simulink model "drone"  (R2019b)
settings: Solver=FixedStepAuto  StartTime=0.0  StopTime=10.0  FixedStep=0.5  RelTol=1e-3
model workspace (MAT data in the model file):
  UAVid = 0
undefined symbols (not defined in the file or in its folder): m, n
libraries: aerolibactuator x3
settings Model: ParameterArgumentNames=UAVid  OrderedModelArguments=off  Creator=Rafael.Casado  LastModifiedBy=paloma

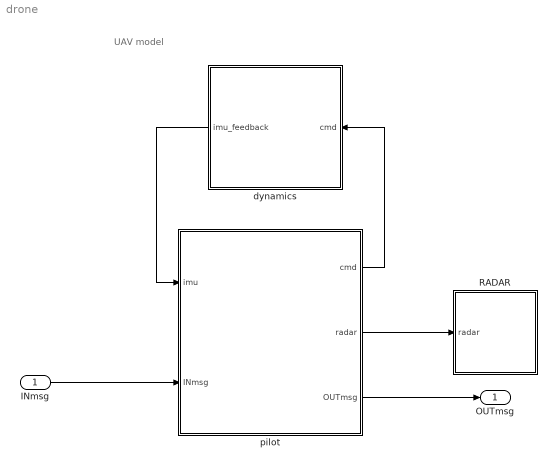
== system drone ==
  note: UAV model
  INmsg : Inport  OutputPortMessageModes=m  OutDataTypeStr=Bus: bus_msg  BusOutputAsStruct=on
  RADAR : Subsystem
      mask Display:
      | plot([00 10], [05 05])
      | plot([05 05], [00 10])
      | 
      | plot([01 09 09 01 01], [01 01 09 09 01])
      | plot([03 07 07 03 03], [03 03 07 07 03])
  dynamics : Subsystem
  pilot : Stateflow chart  TreatAsAtomicUnit=on
  OUTmsg : Outport  OutDataTypeStr=Bus: bus_msg  BusOutputAsStruct=on
  wires:
  pilot/2(radar) -> RADAR/1(radar)
  INmsg/1 -> pilot/2(INmsg)
  pilot/1(cmd) -> dynamics/1(cmd)
  pilot/3(OUTmsg) -> OUTmsg/1
  dynamics/1(imu_feedback) -> pilot/1(imu)

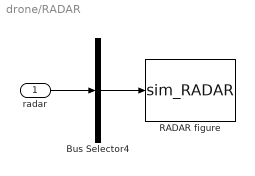
== system drone/RADAR ==
  radar : Inport
  Bus Selector4 : BusSelector  OutputSignals=id,x,y,z  OutputAsBus=on
  RADAR figure : MATLABFcn  StartFcn=|  MATLABFcn=sim_RADAR  OutputDimensions=0  Output1D=off
      | clear functions;
      | clc;
      mask Display: patch([50 -50 -50 50], [40 40 -60 -60], [1 1 1])
  wires:
  radar/1 -> Bus Selector4/1
  Bus Selector4/1 -> RADAR figure/1

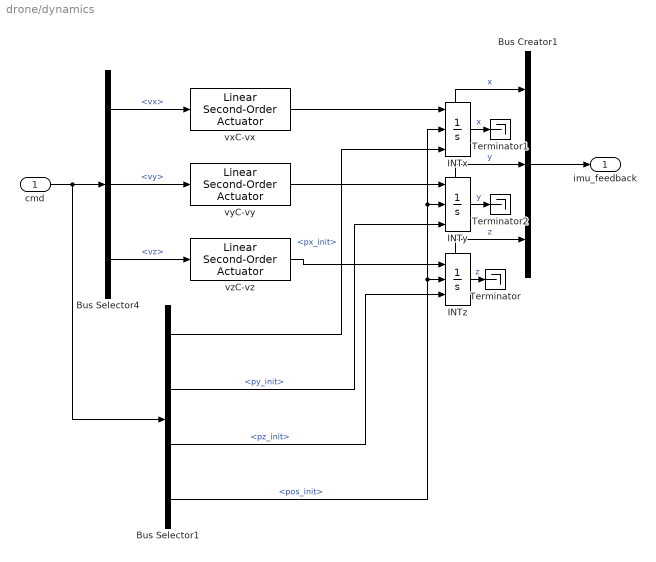
== system drone/dynamics ==
  cmd : Inport
  Bus Creator1 : BusCreator  Inputs=3  OutDataTypeStr=Bus: bus_IMU
      settings: InheritFromInputs=off
  Bus Selector1 : BusSelector  OutputSignals=px_init,py_init,pz_init,pos_init
  Bus Selector4 : BusSelector  OutputSignals=vx,vy,vz
  INTx : Integrator  ExternalReset=rising  InitialConditionSource=external  ShowStatePort=on
  INTy : Integrator  ExternalReset=rising  InitialConditionSource=external  ShowStatePort=on
  INTz : Integrator  ExternalReset=rising  InitialConditionSource=external  ShowStatePort=on
  Terminator : Terminator
  Terminator1 : Terminator
  Terminator2 : Terminator
  vxC-vx : aerolibactuator/Linear Second-Order Actuator  wn_fin=1  z_fin=0.3  fin_act_0=0  fin_act_vel=0
      settings: SourceProductName=Aerospace Blockset  SourceProductBaseCode=AE
  vyC-vy : aerolibactuator/Linear Second-Order Actuator  wn_fin=1  z_fin=0.3  fin_act_0=0  fin_act_vel=0
      settings: SourceProductName=Aerospace Blockset  SourceProductBaseCode=AE
  vzC-vz : aerolibactuator/Linear Second-Order Actuator  wn_fin=1  z_fin=0.3  fin_act_0=0  fin_act_vel=0
      settings: SourceProductName=Aerospace Blockset  SourceProductBaseCode=AE
  imu_feedback : Outport  SourceOfInitialOutputValue=Input signal  OutputWhenDisabled=reset  VectorParamsAs1DForOutWhenUnconnected=off
  wires:
  Bus Creator1/1 -> imu_feedback/1
  INTy/State -> Bus Creator1/2  "y"
  INTx/State -> Bus Creator1/1  "x"
  INTz/State -> Bus Creator1/3  "z"
  Bus Selector4/3 -> vzC-vz/1  "<vz>"
  Bus Selector4/1 -> vxC-vx/1  "<vx>"
  Bus Selector4/2 -> vyC-vy/1  "<vy>"
  vxC-vx/1 -> INTx/1
  vyC-vy/1 -> INTy/1
  vzC-vz/1 -> INTz/1
  Bus Selector1/1 -> INTx/3  "<px_init>"
  Bus Selector1/4 -> INTz/2, INTy/2, INTx/2  "<pos_init>"
  Bus Selector1/2 -> INTy/3  "<py_init>"
  cmd/1 -> Bus Selector1/1, Bus Selector4/1
  Bus Selector1/3 -> INTz/3  "<pz_init>"
  INTz/1 -> Terminator/1  "z"
  INTy/1 -> Terminator2/1  "y"
  INTx/1 -> Terminator1/1  "x"

== stateflow chart drone/pilot ==
  state NAVIGATOR [parallel]
    settings: executionOrder=1
    state INIT
      entry:
      initF
    state IDLE
      entry:
      idleF
    state TAKINGOFF
      entry:
      takingoffF
    state LANDING
      entry,during:
      landingF
    state FLYING
      entry, during:
      d = flyingF;
    (default) -> INIT
    INIT -> IDLE : [active]
    IDLE -> TAKINGOFF : [delivering]
    LANDING -> IDLE : [imu.z < 1]
    TAKINGOFF -> FLYING : [imu.z > 20]
    FLYING -> LANDING : [d<10]
  state COMUNICATIONS [parallel]
    updateRadar
    msgsProcess
    settings: executionOrder=2
    state msgsProcess [function]
      (default) -> (junction 143)
      (junction 143) -> (junction 138) [order 1] : INmsg
      (junction 145) -> (junction 143)
      (junction 143) -> (junction 139) [order 2]
      (junction 138) -> (junction 145) : {UAVmsgProcess}
  data: dis function_output; imu input Bus: bus_IMU; cmd output Bus: bus_command; INmsg input Bus: bus_msg; radar output Bus: bus_radar; OUTmsg output Bus: bus_msg; UAVid parameter double; delivering local boolean =false; deliverPos local; curTime local; d local; vto local =1; active local boolean =false
  function initF:
    | function initF
    | 
    | % Leo matriz de posiciones inicio UAVs (*AppDesign)
    | coder.extrinsic('evalin')
    | beginning = evalin('base','R2');
    | len = double(0);
    | len = length(beginning);
    | 
    | %Asigno posiciones de inicio 
    | if UAVid<=len
    |     active = true;
    |     cmd.pos_init = true;
    |     cmd.px_init  = beginning(UAVid,1);
    |     cmd.py_init  = beginning(UAVid,2);
    |     cmd.pz_init  = 0;
    |     
    |     cmd.vx = 0;
    |     cmd.vy = 0;
    |     cmd.vz = 0;
    | end
  function idleF:
    | function idleF
    | 
    | fprintf('%4.1f: drone %.0f en suelo\n',curTime,UAVid);
    | 
    | cmd.pos_init = false;
    | cmd.px_init  = 0;
    | cmd.py_init  = 0;
    | cmd.pz_init  = 0;
    | 
    | % paro motores
    | cmd.vx = 0;
    | cmd.vy = 0;
    | cmd.vz = 0;
    | delivering = false;
    | 
    | % Enviamos mensaje de delivering
    | OUTmsg.data.available = delivering;
    | OUTmsg.data.id = UAVid;
  function takingoffF:
    | function takingoffF
    | 
    | fprintf('%4.1f: drone %.0f despegando\n',curTime,UAVid);
    | 
    | cmd.vz = vto; %asciendo a velocidad asignada a varible vto = 1 m/s
    | 
    | 
    | %Envio mensaje delivering
    | OUTmsg.data.available = delivering;
    | OUTmsg.data.id = UAVid;
  function landingF:
    | function landingF
    | %fprintf('%4.0f: drone %.0f aterrizando\n',curTime,UAVid);
    | 
    | 
    | cmd.vx = 0;
    | cmd.vy = 0;
    | 
    | 
    | if     imu.z > 10
    |        cmd.vz = -2; %m/s
    | elseif imu.z > 4
    |        cmd.vz = -1; %m/s
    | else
    |        cmd.vz = -0.5; %m/s
    | end
  function dis = flyingF:
    | function dis = flyingF
    | 
    | % fprintf('%4.1f: drone %.0f volando hacia (%.0f %.0f)\n'   ...
    | %      ,curTime,UAVid  ...
    | %      ,deliverPos(1),deliverPos(2));
    | 
    | 
    | vel = deliverPos - [imu.x imu.y];
    | dis = norm(vel);
    | vel = vel / dis * 5;
    | 
    | cmd.vx = vel(1);
    | cmd.vy = vel(2);
    | cmd.vz = 0;
  function updateRadar:
    | function updateRadar
    | 
    | coder.extrinsic('get_param')
    | curTime = get_param('simulator','SimulationTime');
    | 
    | radar.id  = UAVid;
    | radar.x = imu.x;
    | radar.y = imu.y;
    | radar.z = imu.z;
    | 
    | % Actualizo informacion que transmito
    | 
    | OUTmsg.data.x = imu.x;
    | OUTmsg.data.y = imu.y;
    | OUTmsg.data.z = imu.z;
    | 
    | OUTmsg.data.vx = cmd.vx;
    | OUTmsg.data.vy = cmd.vy;
    | OUTmsg.data.vz = cmd.vz;
    | 
    | send(OUTmsg);
  function UAVmsgProcess:
    | function UAVmsgProcess
    | 
    | % extraigo informacion del mensaje
    | msg = INmsg.data;
    | discard(INmsg)
    | 
    | %% tratamiento del mensaje
    | 
    | if UAVid == msg.id 
    |     % El mensaje es para mi
    |     if msg.senderATC
    |         %este es un mensaje del ATC para mi
    |         fprintf('%4.1f: drone %.0f recibe una orden de entrega en (%.0f %.0f)\n'   ...
    |              ,curTime,UAVid  ...
    |              ,msg.x,msg.y);
    | 
    |         delivering = true;
    |         deliverPos = [msg.x msg.y];
    |     else
    |         % yo soy el emisor del mensaje
    |         return
    |     end
    | else    
    |     % el mensaje es para otro    
    |     if msg.senderATC
    |         % este es un mensaje del ATC para otro
    |         return
    |     else
    |         % Detección de conflictos
    |         dist = norm([msg.x msg.y msg.z] - [imu.x imu.y imu.z]);
    |         if dist<10
    |             %estamos en conflicto
    | 
    | 
    | 
    | 
    |         end
    | 
    |         
    |     end
    |     
    |     
    |     
    | end
